simulink model "CAT797_lateral_dynamics_backstepping_control"  (R2026a)
settings: Solver=ode4  StopTime=sim_t  FixedStep=0.0001
PreLoadFcn:
  | addpath("G:\Control_Research\Autonomy_Mining_Dump_Truck\src\plant_model\lib")
values from neighbouring files (symbols this model uses):
  C1 = 220.0    [CAT_797F.sldd]
  C2 = 115.0    [CAT_797F.sldd]
  Cf = 5047000.0    [CAT_797F.sldd]
  Cr = 5047000.0    [CAT_797F.sldd]
  Kd = 0.4    [CAT_797F.sldd]
  Lf = 2.5    [CAT_797F.sldd]
  Lr = 2.3    [CAT_797F.sldd]
  Machine_Mass = 280.0    [CAT_797F.sldd]
libraries: simulink_extras x1, lat_dyn_haul_00 x1
settings Model: DataDictionary=CAT_797F.sldd  Creator=marti343  LastModifiedBy=USER
settings OptimizationCC: EnableMemcpy=off
settings HardwareCC: ProdBitPerChar=16.0  ProdBitPerInt=16.0  ProdLargestAtomicInteger=Integer  ProdWordSize=16.0  ProdHWDeviceType=Texas Instruments->C2000
settings RTWCC: GenerateReport=on  LaunchReport=on
settings CodeAppCC: MATLABSourceComments=on

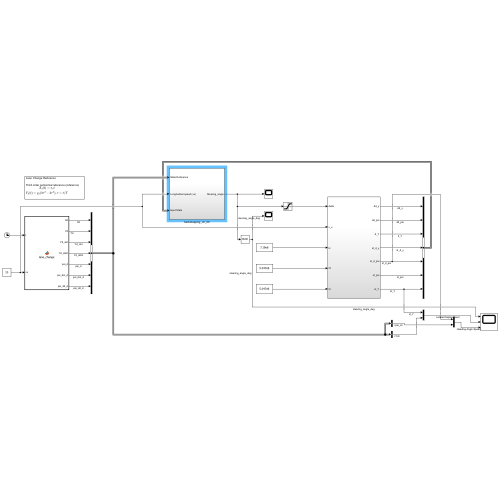
[thumbnail: Simulink's stored preview of the top-level diagram]
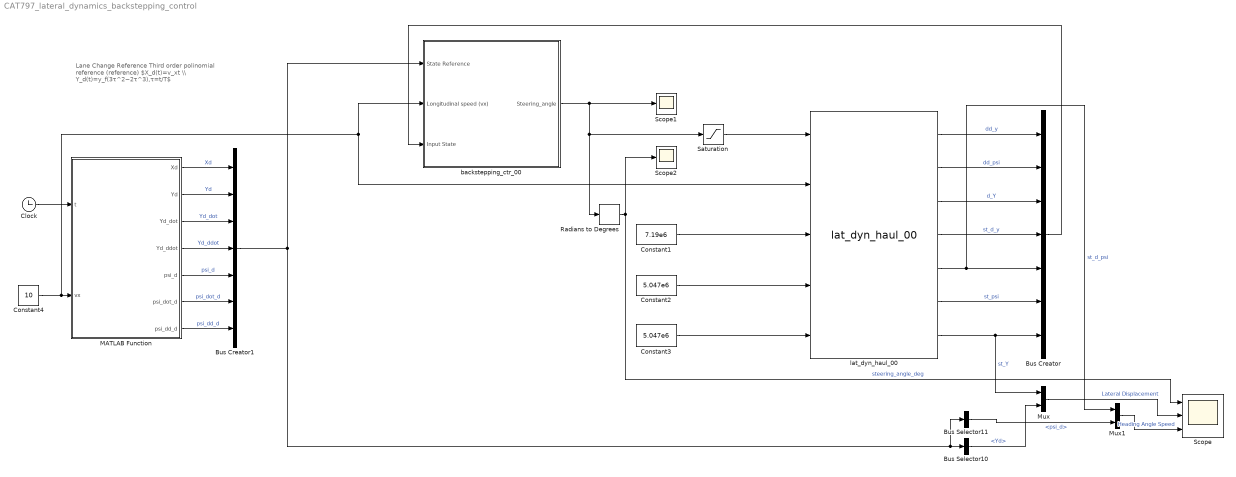
== system CAT797_lateral_dynamics_backstepping_control ==
  note: Lane Change Reference
      |
      | Third order polinomial reference (reference)
      | $X_d​(t)=v_x​t \\ Y_d(t)=y_f(3τ^2−2τ^3),τ=t/T$
  Bus Creator : BusCreator  Inputs=7
  Bus Creator1 : BusCreator  Inputs=7
  Bus Selector10 : BusSelector  OutputSignals=Yd
  Bus Selector11 : BusSelector  OutputSignals=psi_d
  Clock : Clock
  Constant1 : Constant  Value=7.19e6
  Constant2 : Constant  Value=5.047e6
  Constant3 : Constant  Value=5.047e6
  Constant4 : Constant  Value=10
  MATLAB Function : MATLAB Function  TreatAsAtomicUnit=on
  Mux : Mux  Inputs=2
  Mux1 : Mux  Inputs=2
  Radians to Degrees : simulink_extras/Transformations/Radians to Degrees
  Saturation : Saturate  UpperLimit=25  LowerLimit=-25
  Scope : Scope  NumInputPorts=3
      settings: ActiveDisplayString=3  ActiveDisplayYMinimum=-0.012684501332958835  ActiveDisplayYMaximum=0.060865015640720929
  Scope1 : Scope
      settings: ActiveDisplayYMinimum=-1  ActiveDisplayYMaximum=1
  Scope2 : Scope
      settings: ActiveDisplayYMinimum=-1  ActiveDisplayYMaximum=1  DataLoggingVariableName=ScopeData2
  backstepping_ctr_00 : Subsystem
  lat_dyn_haul_00 : lat_dyn_haul_00/lat_dyn_haul_00  SystemSampleTime=-1  VariantActivationTime=update diagram  EmptyChoice=off  PassThrough=off  PassThroughVariantControl=(default)  EmptyChoiceVariantControl=(default)  AllowFlexibleInterface=on  Latency=0  AutoFrameSizeCalculation=off
  wires:
  lat_dyn_haul_00/1 -> Bus Creator/1  "dd_y"
  lat_dyn_haul_00/3 -> Bus Creator/3  "d_Y"
  lat_dyn_haul_00/4 -> Bus Creator/4  "st_d_y"
  Constant4/1 -> lat_dyn_haul_00/2, backstepping_ctr_00/2(Longitudinal speed (vx)), MATLAB Function/2(vx)
  Constant1/1 -> lat_dyn_haul_00/3
  Constant2/1 -> lat_dyn_haul_00/4
  Constant3/1 -> lat_dyn_haul_00/5
  Saturation/1 -> lat_dyn_haul_00/1
  lat_dyn_haul_00/2 -> Bus Creator/2  "dd_psi"
  lat_dyn_haul_00/6 -> Bus Creator/6  "st_psi"
  lat_dyn_haul_00/7 -> Mux/1, Bus Creator/7  "st_Y"
  Clock/1 -> MATLAB Function/1(t)
  MATLAB Function/1(Xd) -> Bus Creator1/1  "Xd"
  MATLAB Function/2(Yd) -> Bus Creator1/2  "Yd"
  MATLAB Function/5(psi_d) -> Bus Creator1/5  "psi_d"
  MATLAB Function/6(psi_dot_d) -> Bus Creator1/6  "psi_dot_d"
  MATLAB Function/7(psi_dd_d) -> Bus Creator1/7  "psi_dd_d"
  Bus Creator1/1 -> backstepping_ctr_00/1(State Reference), Bus Selector11/1, Bus Selector10/1
  Bus Selector10/1 -> Mux/2  "<Yd>"
  Bus Selector11/1 -> Mux1/2  "<psi_d>"
  lat_dyn_haul_00/5 -> Bus Creator/5, Mux1/1  "st_d_psi"
  Bus Creator/1 -> backstepping_ctr_00/3(Input State)
  backstepping_ctr_00/1(Steering_angle) -> Scope1/1, Saturation/1, Radians to Degrees/1
  Radians to Degrees/1 -> Scope/1, Scope2/1  "steering_angle_deg"
  Mux/1 -> Scope/2  "Lateral Displacement"
  Mux1/1 -> Scope/3  "Heading Angle Speed"
  MATLAB Function/3(Yd_dot) -> Bus Creator1/3  "Yd_dot"
  MATLAB Function/4(Yd_ddot) -> Bus Creator1/4  "Yd_ddot"

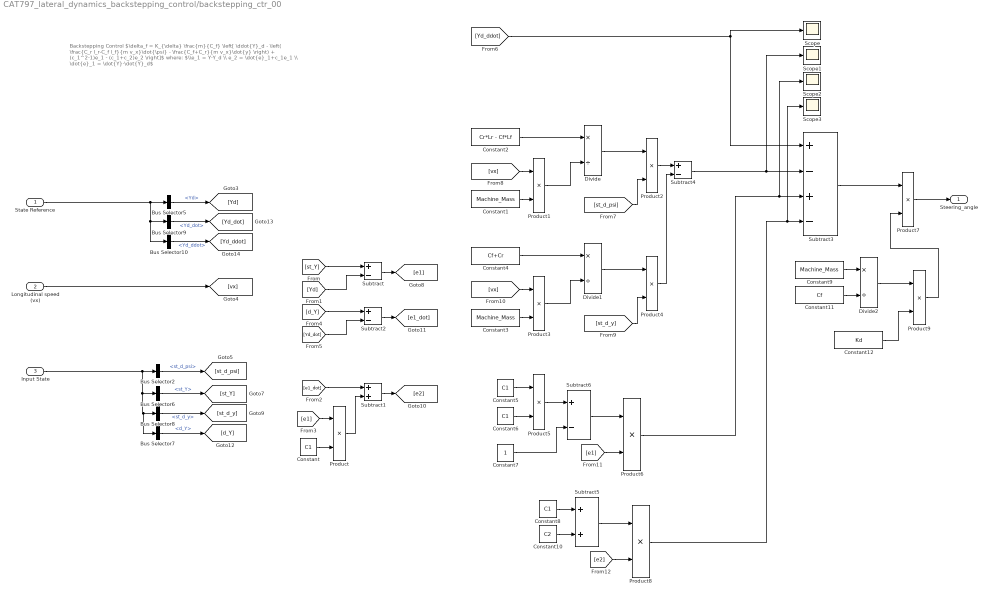
== system CAT797_lateral_dynamics_backstepping_control/backstepping_ctr_00 ==
  note: Backstepping Control
      |
      | $\delta_f = K_{\delta} \frac{m}{C_f} \left[ \ddot{Y}_d - \left( \frac{C_r l_r-C_f l_f}{m v_x}\dot{\psi} - \frac{C_f+C_r}{m v_x}\dot{y} \right) + (c_1^2-1)e_1 - (c_1+c_2)e_2 \right]$
      |
      | where:
      | $\\e_1 = Y-Y_d \\ e_2 = \dot{e}_1+c_1e_1 \\ \dot{e}_1 = \dot{Y}-\dot{Y}_d$
  State Reference : Inport
  Longitudinal speed (vx) : Inport  Port=2
  Input State : Inport  Port=3
  Bus Selector10 : BusSelector  OutputSignals=Yd_ddot
  Bus Selector2 : BusSelector  OutputSignals=st_d_psi
  Bus Selector5 : BusSelector  OutputSignals=Yd
  Bus Selector6 : BusSelector  OutputSignals=st_Y
  Bus Selector7 : BusSelector  OutputSignals=d_Y
  Bus Selector8 : BusSelector  OutputSignals=st_d_y
  Bus Selector9 : BusSelector  OutputSignals=Yd_dot
  Constant{,5..6,8} (4 alike) : Constant  Value=C1
  Constant1 : Constant  Value=Machine_Mass
  Constant10 : Constant  Value=C2
  Constant11 : Constant  Value=Cf
  Constant12 : Constant  Value=Kd
  Constant2 : Constant  Value=Cr*Lr - Cf*Lf
  Constant3 : Constant  Value=Machine_Mass
  Constant4 : Constant  Value=Cf+Cr
  Constant7 : Constant
  Constant9 : Constant  Value=Machine_Mass
  Divide : Product  Inputs=*/
  Divide1 : Product  Inputs=*/
  Divide2 : Product  Inputs=*/
  Product{,1..9} (10 alike) : Product
  Scope{,1..3} (4 alike) : Scope
      Scope settings: ActiveDisplayYMinimum=-1  ActiveDisplayYMaximum=1  DataLoggingVariableName=ScopeData3
      Scope1 settings: ActiveDisplayYMinimum=-0.31  ActiveDisplayYMaximum=-0.10999999999999999  DataLoggingVariableName=ScopeData4
      Scope2 settings: ActiveDisplayYMinimum=-1  ActiveDisplayYMaximum=1  DataLoggingVariableName=ScopeData5
      Scope3 settings: ActiveDisplayYMinimum=-1  ActiveDisplayYMaximum=1  DataLoggingVariableName=ScopeData6
  Subtract{,2,4,6} (4 alike) : Sum  Inputs=+-
  Subtract1 : Sum
  Subtract3 : Sum  Inputs=+-+-
  Subtract5 : Sum
  Steering_angle : Outport
  wires:
  Bus Selector5/1 -> [Yd]  "<Yd>"
  Bus Selector6/1 -> [st_Y]  "<st_Y>"
  Longitudinal speed (vx)/1 -> [vx]
  Bus Selector2/1 -> [st_d_psi]  "<st_d_psi>"
  Bus Selector8/1 -> [st_d_y]  "<st_d_y>"
  [st_Y] -> Subtract/1
  [Yd] -> Subtract/2
  Subtract/1 -> [e1]
  Subtract1/1 -> [e2]
  Product/1 -> Subtract1/2
  [e1_dot] -> Subtract1/1
  Subtract2/1 -> [e1_dot]
  [Yd_dot] -> Subtract2/2
  [d_Y] -> Subtract2/1
  Input State/1 -> Bus Selector7/1, Bus Selector8/1, Bus Selector6/1, Bus Selector2/1
  Bus Selector7/1 -> [d_Y]  "<d_Y>"
  Bus Selector9/1 -> [Yd_dot]  "<Yd_dot>"
  State Reference/1 -> Bus Selector5/1, Bus Selector9/1, Bus Selector10/1
  Bus Selector10/1 -> [Yd_ddot]  "<Yd_ddot>"
  [e1] -> Product/1
  Constant/1 -> Product/2
  [Yd_ddot] -> Subtract3/1, Scope/1
  [vx] -> Product1/1
  Constant1/1 -> Product1/2
  Product1/1 -> Divide/2
  Constant2/1 -> Divide/1
  Divide/1 -> Product2/1
  [st_d_psi] -> Product2/2
  Product2/1 -> Subtract4/1
  Subtract4/1 -> Scope1/1, Subtract3/2
  [st_d_y] -> Product4/2
  Divide1/1 -> Product4/1
  Constant4/1 -> Divide1/1
  Product3/1 -> Divide1/2
  Constant3/1 -> Product3/2
  [vx] -> Product3/1
  Product4/1 -> Subtract4/2
  Constant5/1 -> Product5/1
  Constant6/1 -> Product5/2
  Product5/1 -> Subtract6/1
  Constant7/1 -> Subtract6/2
  Subtract6/1 -> Product6/1
  [e1] -> Product6/2
  Product6/1 -> Scope2/1, Subtract3/3
  [e2] -> Product8/2
  Subtract5/1 -> Product8/1
  Constant10/1 -> Subtract5/2
  Constant8/1 -> Subtract5/1
  Subtract3/1 -> Product7/1
  Product8/1 -> Scope3/1, Subtract3/4
  Product7/1 -> Steering_angle/1
  Constant9/1 -> Divide2/1
  Constant11/1 -> Divide2/2
  Divide2/1 -> Product9/1
  Product9/1 -> Product7/2
  Constant12/1 -> Product9/2

== matlab function CAT797_lateral_dynamics_backstepping_control/MATLAB Function ==
  data: t input; Xd output; vx input; Yd output; Yd_dot output; Yd_ddot output; psi_d output; psi_dot_d output; psi_dd_d output
function [Xd, Yd, Yd_dot, Yd_ddot, psi_d, psi_dot_d, psi_dd_d] = lane_change(t, vx)

% PARAMETERS (tune these)
T  = 10;       % duration [s]
yf = 3.5;      % lateral shift [m]

% Normalize time
tau = t / T;

% Clamp tau between 0 and 1
if tau > 1
    tau = 1;
end
if tau < 0
    tau = 0;
end

% =========================
% POSITION
% =========================
Xd = vx * t;
Yd = yf * (3*tau^2 - 2*tau^3);

% =========================
% FIRST DERIVATIVE
% =========================
Xd_dot = vx;
Yd_dot = yf * (6*tau/T - 6*tau^2/T);

% =========================
% SECOND DERIVATIVE
% =========================
Xd_ddot = 0;
Yd_ddot = yf * (6/T^2 - 12*tau/T^2);

% =========================
% HEADING
% =========================
psi_d = atan2(Yd_dot, Xd_dot);

% =========================
% YAW RATE
% =========================
psi_dot_d = (Xd_dot * Yd_ddot - Yd_dot * Xd_ddot) / ...
            (Xd_dot^2 + Yd_dot^2);

% =========================
% YAW ACCELERATION (optional)
% =========================
% Numerical approximation (simple)
dt = 1e-3;

tau2 = (t+dt)/T;
if tau2 > 1
    tau2 = 1;
end

Yd_dot_2 = yf * (6*tau2/T - 6*tau2^2/T);
psi_d_2 = atan2(Yd_dot_2, vx);

psi_dd_d = (psi_d_2 - psi_d) / dt;

end
